simulink library "Mechanical_Library"  (R2020b)
settings: Solver=ode15s  StartTime=0.0  StopTime=10.0  RelTol=1e-3  EnableMultiTasking=on
libraries: fl_lib x2
settings Model: Creator=ssekkai  LastModifiedBy=camka
settings DataIOCC: SaveFormat=Array  ReturnWorkspaceOutputs=off
settings OptimizationCC: LifeSpan=inf
settings DebuggingCC: UnderspecifiedInitializationDetection=Classic  MergeDetectMultiDrivingBlocksExec=none  SolverPrmCheckMsg=warning  SFUnexpectedBacktrackingDiag=warning  SFNoUnconditionalDefaultTransitionDiag=warning  SFExecutionAtInitializationDiag=none  ArithmeticOperatorsInVariantConditions=warning
settings HardwareCC: ProdBitPerPointer=32  ProdBitPerSizeT=32  ProdBitPerPtrDiffT=32  ProdLargestAtomicFloat=None  ProdIntDivRoundTo=Undefined  ProdEndianess=Unspecified  ProdWordSize=32  ProdHWDeviceType=32-bit Generic
settings ModelReferenceCC: PropagateSignalLabelsOutOfModel=off
settings SFSimCC: SimUseLocalCustomCode=off  CustomCodeUndefinedFunction=UseInterfaceOnly
settings RTWCC: RTWUseLocalCustomCode=off
settings CodeAppCC: StateflowObjectComments=on
settings GRTTargetCC: TargetLangStandard=C89/C90 (ANSI)
settings ConfigComp: CovMetricSettings=dw  CovSaveCumulativeToWorkspaceVar=on  CovSaveSingleToWorkspaceVar=on  CovExternalEMLEnable=off  CovSFcnEnable=off

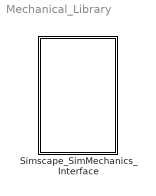
== system Mechanical_Library ==
  Simscape_SimMechanics_Interface : Subsystem

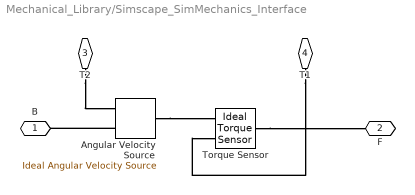
== system Mechanical_Library/Simscape_SimMechanics_Interface ==
  Angular Velocity Source : fl_lib/Mechanical/Mechanical Sources/Ideal Angular Velocity Source
  Torque Sensor : fl_lib/Mechanical/Mechanical Sensors/Ideal Torque Sensor
  B : PMIOPort  Side=Left
  F : PMIOPort  Port=2  Side=Left
  T2 : PMIOPort  Port=3  Side=Left
  T1 : PMIOPort  Port=4  Side=Right
  connections:
  Angular Velocity Source/LConn1 -- Torque Sensor/RConn1
  T2/RConn1 -- Angular Velocity Source/RConn1
  Angular Velocity Source/RConn2 -- B/RConn1
  T1/RConn1 -- Torque Sensor/RConn2
  Torque Sensor/LConn1 -- F/RConn1
